simulink model "PositionControl"  (R2023a)
settings: Solver=FixedStepAuto  StartTime=0.0  StopTime=4  FixedStep=Ts  RelTol=1e-3
values from neighbouring files (symbols this model uses):
  refx = 10*rand-5    [RunPositionControl.m]    (also in RunPositionControlNet.m = 2; parte2_apartado_i.m = valores_refx(i))
  refy = 10*rand-5    [RunPositionControl.m]    (also in RunPositionControlNet.m = 2; parte2_apartado_i.m = valores_refy(j))
  Ts = 100e-3    (= 0.1)    [RunPositionControl.m]    (also in RunPositionControlNet.m; parte2_apartado_i.m)
undefined symbols (not defined in the file or in its folder): DiscIntNeverNeededParam
settings Model: Creator=Edu  LastModifiedBy=micue
settings DataIOCC: ReturnWorkspaceOutputs=off

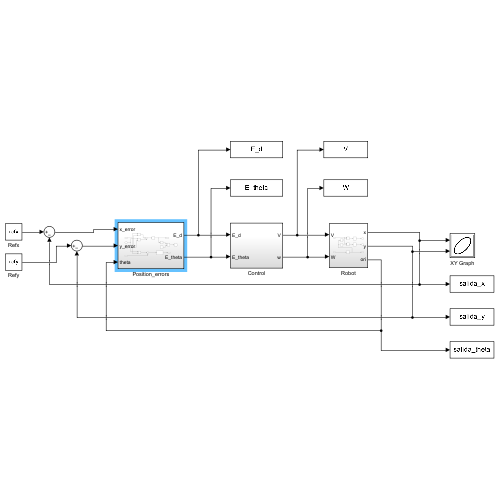
[thumbnail: Simulink's stored preview of the top-level diagram]
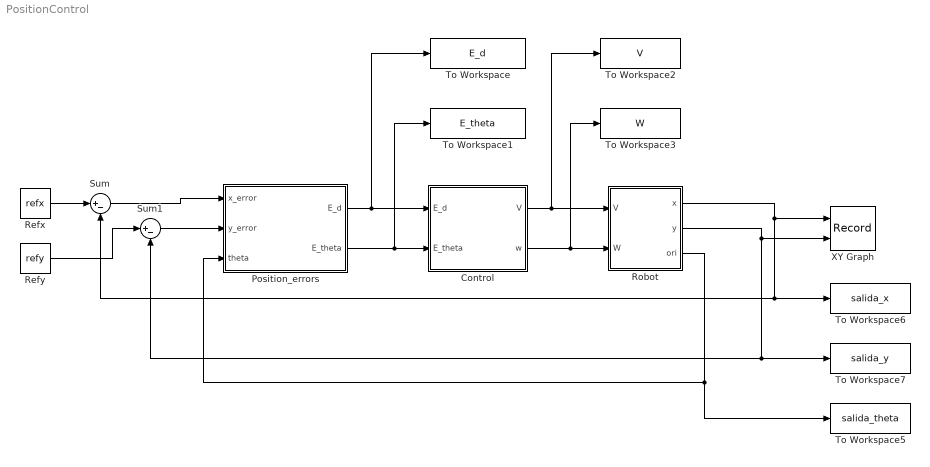
== system PositionControl ==
  Control : Subsystem
  Position_errors : Subsystem
  Refx : Constant  Value=refx
  Refy : Constant  Value=refy
  Robot : Subsystem
  Sum : Sum  Inputs=|+-
  Sum1 : Sum  Inputs=|+-
  To Workspace : ToWorkspace  VariableName=E_d  SaveFormat=Structure With Time  SampleTime=-1
  To Workspace1 : ToWorkspace  VariableName=E_theta  SaveFormat=Structure With Time  SampleTime=-1
  To Workspace2 : ToWorkspace  VariableName=V  SaveFormat=Structure With Time  SampleTime=-1
  To Workspace3 : ToWorkspace  VariableName=W  SaveFormat=Structure With Time  SampleTime=-1
  To Workspace5 : ToWorkspace  VariableName=salida_theta  SaveFormat=Structure With Time  SampleTime=-1
  To Workspace6 : ToWorkspace  VariableName=salida_x  SaveFormat=Structure With Time  SampleTime=-1
  To Workspace7 : ToWorkspace  VariableName=salida_y  SaveFormat=Structure With Time  SampleTime=-1
  XY Graph : Record  FileSettingsInternal="{\"entries\":[{\"content\":{\"excelSettings\":{\"content\":{},\"type\":\"Streamout.ExcelSettings\"}},\"type\":\"Streamout.FileSettingStorage\",\"uuid\":\"\"}],\"packageUris\":[\"http:\\/\\/schema.mathworks.com\\/mf0\\/streamout_blocks\\/R2020a\"],\"version\":\"1.0\"}"  Layout=[1 1]  SignalsInternal="{\"entries\":[{\"content\":{\"signals\":[{\"content\":{\"blockPath\":[],\"dimensions\":[1],\"domain\":\"\",\"lineColor\":\"#a2142f\",\"plots\":[1],\"port\":1,\"sid\":[\"\"],\"signalID\":14542,\"signalName\":\"Robot:1\"},\"type\":\"RecordBlkView.Signal\",\"uuid\":\"\"},{\"content\":{\"blockPath\":[],\"dimensions\":[1],\"domain\":\"\",\"lineColor\":\"#139fff\",\"plots\":[1],\"port\":2,\"sid\":[\"\"],\"signalID\":14546,\"signalName\":\"Robot:2\"},\"type\":\"RecordBlkView.Signal\",\"uuid\":\"\"}]},\"type\":\"RecordBlkView.InputSignals\",\"uuid\":\"\"}],\"packageUris\":[\"http:\\/\\/schema.mathworks.com\\/mf0\\/streamout_blocks\\/R2020a\"],\"version\":\"1.0\"}"  VisualizationBindings="{\"xyplotplugin\":{\"info\":[{\"series\":[{\"bindingParametersList\":[{\"parameter\":\"X-Axis\",\"signalID\":14542,\"signalName\":\"Robot:1\"},{\"parameter\":\"Y-Axis\",\"signalID\":14546,\"signalName\":\"Robot:2\"}],\"seriesID\":37301}],\"subplotID\":1}]}}"  CompatibilityTag=XY
  wires:
  Position_errors/2(E_theta) -> To Workspace1/1, Control/2(E_theta)
  Refy/1 -> Sum1/1
  Refx/1 -> Sum/1
  Control/1(V) -> To Workspace2/1, Robot/1(V)
  Position_errors/1(E_d) -> Control/1(E_d), To Workspace/1
  Robot/2(y) -> To Workspace7/1, Sum1/2, XY Graph/2
  Robot/3(ori) -> To Workspace5/1, Position_errors/3(theta)
  Control/2(w) -> To Workspace3/1, Robot/2(W)
  Sum/1 -> Position_errors/1(x_error)
  Sum1/1 -> Position_errors/2(y_error)
  Robot/1(x) -> Sum/2, To Workspace6/1, XY Graph/1

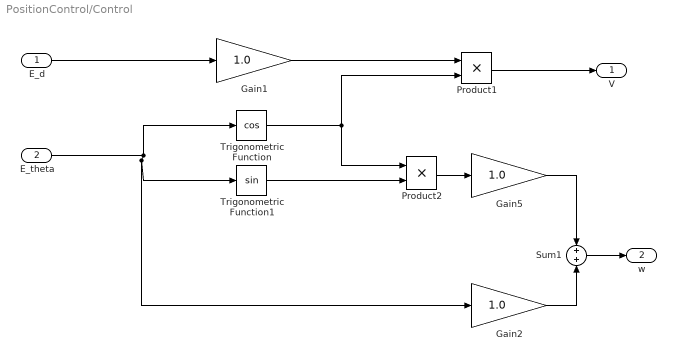
== system PositionControl/Control ==
  E_d : Inport
  E_theta : Inport  Port=2
  Gain1 : Gain  Gain=1.0
  Gain2 : Gain  Gain=1.0
  Gain5 : Gain  Gain=1.0
  Product1 : Product
  Product2 : Product
  Sum1 : Sum
  Trigonometric Function : Trigonometry  Operator=cos
  Trigonometric Function1 : Trigonometry
  V : Outport  VectorParamsAs1DForOutWhenUnconnected=off
  w : Outport  Port=2  VectorParamsAs1DForOutWhenUnconnected=off
  wires:
  E_theta/1 -> Trigonometric Function/1, Trigonometric Function1/1, Gain2/1
  E_d/1 -> Gain1/1
  Trigonometric Function/1 -> Product1/2, Product2/1
  Product1/1 -> V/1
  Trigonometric Function1/1 -> Product2/2
  Product2/1 -> Gain5/1
  Gain1/1 -> Product1/1
  Gain5/1 -> Sum1/1
  Gain2/1 -> Sum1/2
  Sum1/1 -> w/1

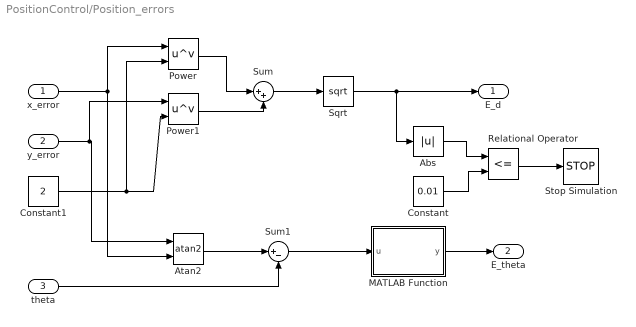
== system PositionControl/Position_errors ==
  x_error : Inport
  y_error : Inport  Port=2
  theta : Inport  Port=3
  Abs : Abs  SaturateOnIntegerOverflow=off
  Atan2 : Trigonometry  Operator=atan2
  Constant : Constant  Value=0.01
  Constant1 : Constant  Value=2
  MATLAB Function : MATLAB Function  TreatAsAtomicUnit=on
  Power : Math  Operator=pow
  Power1 : Math  Operator=pow
  Relational Operator : RelationalOperator  Operator=<=  OutDataTypeStr=boolean  RndMeth=Simplest  InputSameDT=off
  Sqrt : Sqrt
  Stop Simulation : Stop
  Sum : Sum  Inputs=|++
  Sum1 : Sum  Inputs=|+-
  E_d : Outport
  E_theta : Outport  Port=2
  wires:
  x_error/1 -> Atan2/2, Power/1
  y_error/1 -> Atan2/1, Power1/1
  Sum/1 -> Sqrt/1
  Sqrt/1 -> Abs/1, E_d/1
  Atan2/1 -> Sum1/1
  theta/1 -> Sum1/2
  Sum1/1 -> MATLAB Function/1(u)
  Relational Operator/1 -> Stop Simulation/1
  Abs/1 -> Relational Operator/1
  Constant/1 -> Relational Operator/2
  MATLAB Function/1(y) -> E_theta/1
  Constant1/1 -> Power/2, Power1/2
  Power1/1 -> Sum/2
  Power/1 -> Sum/1

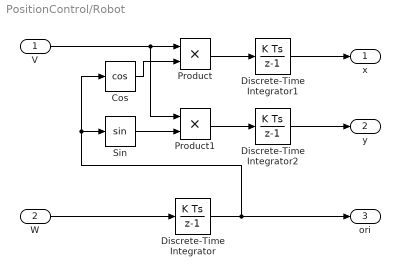
== system PositionControl/Robot ==
  V : Inport
  W : Inport  Port=2
  Cos : Trigonometry  Operator=cos
  Discrete-Time Integrator : DiscreteIntegrator  SampleTime=Ts  ICPrevOutput=DiscIntNeverNeededParam  ICPrevScaledInput=DiscIntNeverNeededParam
  Discrete-Time Integrator1 : DiscreteIntegrator  SampleTime=Ts  ICPrevOutput=DiscIntNeverNeededParam  ICPrevScaledInput=DiscIntNeverNeededParam
  Discrete-Time Integrator2 : DiscreteIntegrator  SampleTime=Ts  ICPrevOutput=DiscIntNeverNeededParam  ICPrevScaledInput=DiscIntNeverNeededParam
  Product : Product
  Product1 : Product
  Sin : Trigonometry
  x : Outport
  y : Outport  Port=2
  ori : Outport  Port=3
  wires:
  Discrete-Time Integrator/1 -> ori/1, Sin/1, Cos/1
  Discrete-Time Integrator1/1 -> x/1
  Cos/1 -> Product/2
  V/1 -> Product1/1, Product/1
  Sin/1 -> Product1/2
  Discrete-Time Integrator2/1 -> y/1
  W/1 -> Discrete-Time Integrator/1
  Product1/1 -> Discrete-Time Integrator2/1
  Product/1 -> Discrete-Time Integrator1/1

== matlab function PositionControl/Position_errors/MATLAB Function ==
  data: u input; y output
function y = tranformar(u)

y = wrapTo180(u);
